simulink model "nav_leha19b"  (R2019b)
settings: Solver=FixedStepDiscrete  StartTime=0.0  StopTime=2500  FixedStep=dT  RelTol=1e-3
values from neighbouring files (symbols this model uses):
  al_gp_M = k    (= 2)    [gnss_data_orig.m]
  al_gp_max = 15    [model_nav_system_flight_simulation_orig.m]
  al_gp_mu = 3.986004418E+14    (= 398600441800000)    [gnss_data_orig.m]
  al_gp_resolution = 1000    [gnss_data_orig.m]
  al_gp_t0 = gnss_strings_2(1,4)    [gnss_data_orig.m]
  dT = 1    [model_nav_system_flight_simulation_orig.m]
  mean_p_ion = 1.3    [model_nav_system_flight_simulation_orig.m]
  mean_p_trop = 0.3    [model_nav_system_flight_simulation_orig.m]
  P0_b_g = zeros(23,23)    [model_nav_system_flight_simulation_orig.m]
  P_b = zeros(21, 21)    [model_nav_system_flight_simulation_orig.m]
  R_a = 6378136    [model_nav_system_flight_simulation_orig.m]
  R_betta = 0.0053171    [model_nav_system_flight_simulation_orig.m]
  R_betta1 = 71 * 10^-7    (= 7.1e-06)    [model_nav_system_flight_simulation_orig.m]
  R_e2 = 0    [model_nav_system_flight_simulation_orig.m]
  R_ge = 9.78049    [model_nav_system_flight_simulation_orig.m]
  R_q = 0.00346775    [model_nav_system_flight_simulation_orig.m]
  R_u = 7.292115*10^(-5)    (= 7.292115e-05)    [model_nav_system_flight_simulation_orig.m]
  sigma_error_acs0 = [SKO_del_n_x SKO_del_n_y SKO_del_n_z]    [model_nav_system_flight_simulation_orig.m]
  sigma_error_DUS0 = [SKO_del_Omega_x SKO_del_Omega_y SKO_del_Omega_z]    [model_nav_system_flight_simulation_orig.m]
  sigma_gnss0 = SKO_p_del_T + SKO_p_del_t + mean_p_ion + mean_p_trop + SKO_p_mnogoluch + SKO_p_noise    (= 5.61)    [model_nav_system_flight_simulation_orig.m]
  SKO_p_del_T = 3    [model_nav_system_flight_simulation_orig.m]
  SKO_p_del_t = 0.01    [model_nav_system_flight_simulation_orig.m]
  SKO_p_mnogoluch = 0.5    [model_nav_system_flight_simulation_orig.m]
  SKO_p_noise = 0.5    [model_nav_system_flight_simulation_orig.m]
  tr_H = flight_mission(3,1)    [model_nav_system_flight_simulation_orig.m]
  W = W'    [model_nav_system_flight_simulation_orig.m]
  X0 = X0'    [model_nav_system_flight_simulation_orig.m]
  X0_b_g = X0_b_g * 0    [model_nav_system_flight_simulation_orig.m]
undefined symbols (not defined in the file or in its folder): al_gp_e, al_gp_health, al_gp_i, al_gp_lan, al_gp_m0, al_gp_sqrt_a, al_gp_w, sigma_error_D_p, sigma_error_D_p1, sigma_gnss0_0, tr_course, tr_fi, tr_la, tr_pitch, tr_roll, tr_V_E, tr_V_H, tr_V_N, tr_X_dgsk, tr_Y_dgsk, tr_Z_dgsk
libraries: simulink_extras x8
(part 1 of 3)
settings Model: PacingRate=11  Creator=Алексей  LastModifiedBy=ssa33
settings DebuggingCC: ReadBeforeWriteMsg=DisableAll  WriteAfterWriteMsg=DisableAll  WriteAfterReadMsg=DisableAll  MultiTaskDSMMsg=none  ArithmeticOperatorsInVariantConditions=warning
settings ModelReferenceCC: UpdateModelReferenceTargets=IfOutOfDate
settings SFSimCC: SFSimEcho=off  CustomCodeUndefinedFunction=UseInterfaceOnly

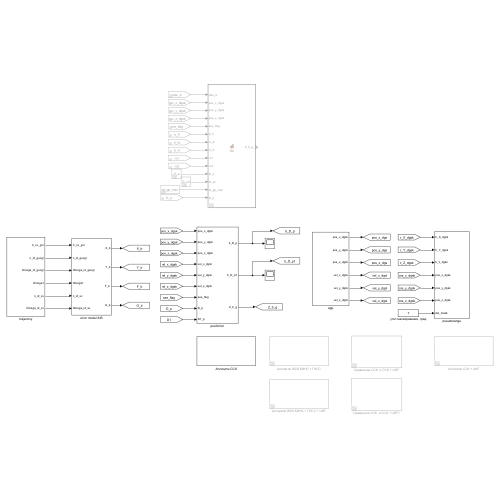
[thumbnail: Simulink's stored preview of the top-level diagram]
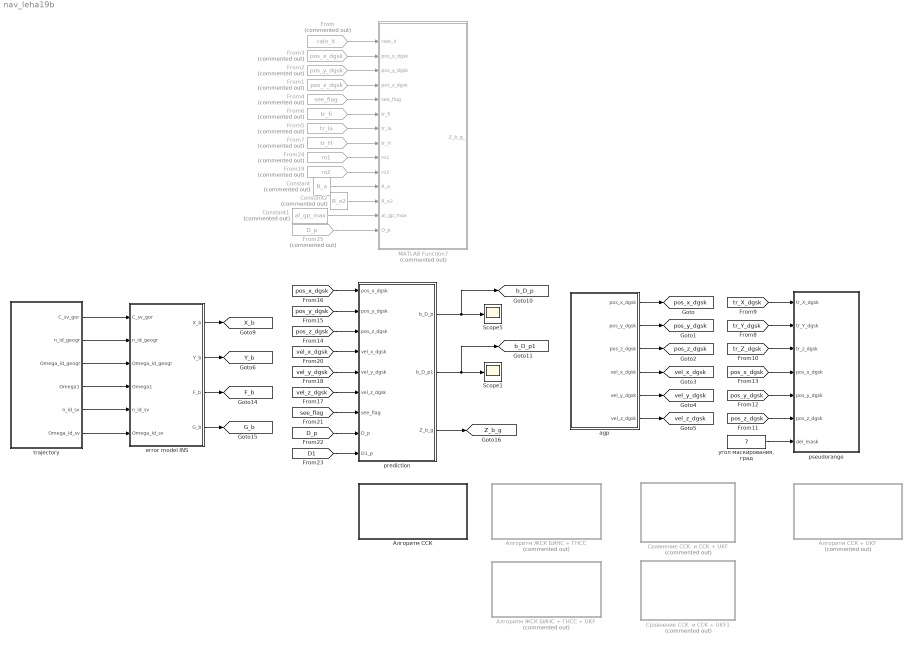
== system nav_leha19b ==
  Constant : Constant  Commented=on  Value=R_a
  Constant1 : Constant  Commented=on  Value=al_gp_max
  Constant2 : Constant  Commented=on  Value=R_e2
  From : From  Commented=on  GotoTag=rate_X  TagVisibility=global
  From1 : From  Commented=on  GotoTag=pos_z_dgsk  TagVisibility=global
  From19 : From  Commented=on  GotoTag=ro2  TagVisibility=global
  From2 : From  Commented=on  GotoTag=pos_y_dgsk  TagVisibility=global
  From24 : From  Commented=on  GotoTag=ro1  TagVisibility=global
  From25 : From  Commented=on  GotoTag=D_p  TagVisibility=global
  From3 : From  Commented=on  GotoTag=pos_x_dgsk  TagVisibility=global
  From4 : From  Commented=on  GotoTag=see_flag  TagVisibility=global
  From5 : From  Commented=on  GotoTag=tr_la  TagVisibility=global
  From6 : From  Commented=on  GotoTag=tr_fi  TagVisibility=global
  From7 : From  Commented=on  GotoTag=tr_H  TagVisibility=global
  MATLAB Function7 : MATLAB Function  Commented=on  TreatAsAtomicUnit=on
  Scope1 : Scope
  Scope5 : Scope
  agp : Subsystem
  error model INS : Subsystem
  "prediction " : Subsystem
  pseudorange : Subsystem
  trajectory : Subsystem
  Алгоритм ЖСК БИНС + ГНСС : Subsystem  Commented=on
  Алгоритм ЖСК БИНС + ГНСС + UKF : Subsystem  Commented=on
  Алгоритм ССК : Subsystem
  Алгоритм ССК + UKF : Subsystem  Commented=on
  Сравнение ССK  и CCK + UKF : Subsystem  Commented=on
  Сравнение ССK  и CCK + UKF1 : Subsystem  Commented=on
  "угол маскирования, град" : Constant  Value=7
  tag scope: F_b=global, G_b=global, X_b=global, Y_b=global, Z_b_g=global, b_D_p1=global, b_D_p=global, pos_x_dgsk=global, pos_y_dgsk=global, pos_z_dgsk=global, vel_x_dgsk=global, vel_y_dgsk=global, vel_z_dgsk=global
  wires:
  agp/1(pos_x_dgsk) -> [pos_x_dgsk]
  agp/2(pos_y_dgsk) -> [pos_y_dgsk]
  agp/3(pos_z_dgsk) -> [pos_z_dgsk]
  [tr_X_dgsk] -> pseudorange/1(tr_X_dgsk)
  [tr_Y_dgsk] -> pseudorange/2(tr_Y_dgsk)
  [tr_Z_dgsk] -> pseudorange/3(tr_z_dgsk)
  [pos_x_dgsk] -> pseudorange/4(pos_x_dgsk)
  [pos_y_dgsk] -> pseudorange/5(pos_y_dgsk)
  [pos_z_dgsk] -> pseudorange/6(pos_z_dgsk)
  "угол маскирования, град"/1 -> pseudorange/7(del_mask)
  agp/4(vel_x_dgsk) -> [vel_x_dgsk]
  agp/5(vel_y_dgsk) -> [vel_y_dgsk]
  agp/6(vel_z_dgsk) -> [vel_z_dgsk]
  error model INS/2(Y_b) -> [Y_b]
  [pos_x_dgsk] -> "prediction "/1(pos_x_dgsk)
  [pos_z_dgsk] -> "prediction "/3(pos_z_dgsk)
  [pos_y_dgsk] -> "prediction "/2(pos_y_dgsk)
  [vel_y_dgsk] -> "prediction "/5(vel_y_dgsk)
  [vel_z_dgsk] -> "prediction "/6(vel_z_dgsk)
  [vel_x_dgsk] -> "prediction "/4(vel_x_dgsk)
  "prediction "/1(b_D_p) -> [b_D_p], Scope5/1
  "prediction "/2(b_D_p1) -> [b_D_p1], Scope1/1
  [see_flag] -> "prediction "/7(see_flag)
  [D_p] -> "prediction "/8(D_p)
  [D1] -> "prediction "/9(D1_p)
  error model INS/1(X_b) -> [X_b]
  error model INS/3("F_b ") -> [F_b]
  error model INS/4(G_b) -> [G_b]
  trajectory/5(n_id_sv) -> error model INS/5(n_id_sv)
  trajectory/1(C_sv_gor) -> error model INS/1(C_sv_gor)
  trajectory/4(Omega1) -> error model INS/4(Omega1)
  trajectory/6(Omega_id_sv) -> error model INS/6(Omega_id_sv)
  trajectory/2(n_id_geogr) -> error model INS/2(n_id_geogr)
  trajectory/3(Omega_id_geogr) -> error model INS/3(Omega_id_geogr)
  From3/1 -> MATLAB Function7/2(pos_x_dgsk)
  From2/1 -> MATLAB Function7/3(pos_y_dgsk)
  From1/1 -> MATLAB Function7/4(pos_z_dgsk)
  From4/1 -> MATLAB Function7/5(see_flag)
  From6/1 -> MATLAB Function7/6(tr_fi)
  From5/1 -> MATLAB Function7/7(tr_la)
  From7/1 -> MATLAB Function7/8(tr_H)
  From24/1 -> MATLAB Function7/9(ro1)
  From19/1 -> MATLAB Function7/10(ro2)
  Constant/1 -> MATLAB Function7/11(R_a)
  Constant2/1 -> MATLAB Function7/12(R_e2)
  Constant1/1 -> MATLAB Function7/13(al_gp_max)
  From25/1 -> MATLAB Function7/14(D_p)
  From/1 -> MATLAB Function7/1(rate_X)
  "prediction "/3(Z_b_g) -> [Z_b_g]

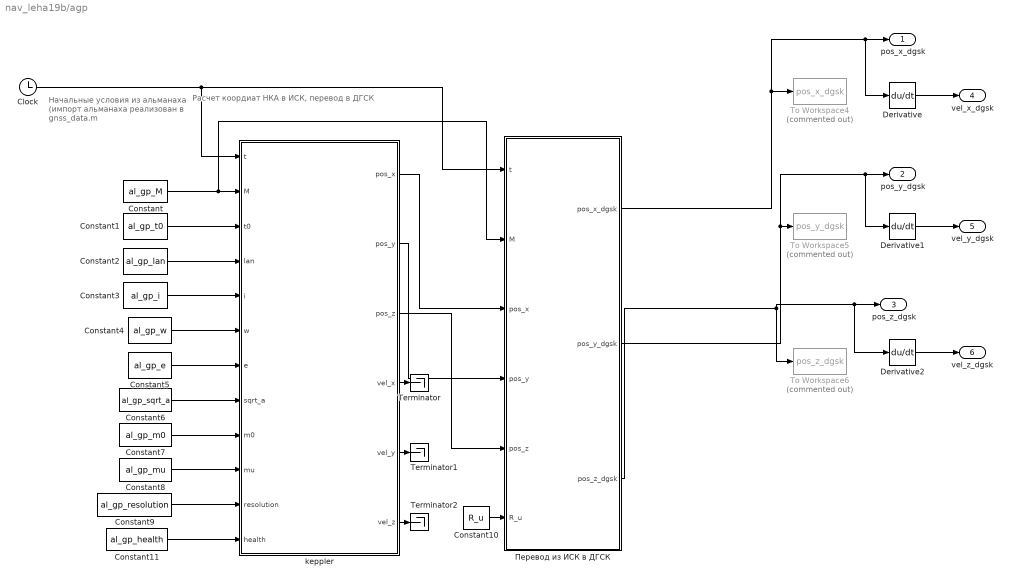
== system nav_leha19b/agp ==
  note: Начальные условия
      | из альманаха
      | (импорт альманаха
      | реализован в gnss_data.m
  note: Расчет коордиат НКА в ИСК, перевод в ДГСК
  Clock : Clock
  Constant : Constant  Value=al_gp_M
  Constant1 : Constant  Value=al_gp_t0
  Constant10 : Constant  Value=R_u
  Constant11 : Constant  Value=al_gp_health
  Constant2 : Constant  Value=al_gp_lan
  Constant3 : Constant  Value=al_gp_i
  Constant4 : Constant  Value=al_gp_w
  Constant5 : Constant  Value=al_gp_e
  Constant6 : Constant  Value=al_gp_sqrt_a
  Constant7 : Constant  Value=al_gp_m0
  Constant8 : Constant  Value=al_gp_mu
  Constant9 : Constant  Value=al_gp_resolution
  Derivative : Derivative
  Derivative1 : Derivative
  Derivative2 : Derivative
  Terminator : Terminator
  Terminator1 : Terminator
  Terminator2 : Terminator
  To Workspace4 : ToWorkspace  Commented=on  VariableName=pos_x_dgsk  SampleTime=-1
      settings: Save2DSignal=2-D array (concatenate along first dimension)
  To Workspace5 : ToWorkspace  Commented=on  VariableName=pos_y_dgsk  SampleTime=-1
      settings: Save2DSignal=2-D array (concatenate along first dimension)
  To Workspace6 : ToWorkspace  Commented=on  VariableName=pos_z_dgsk  SampleTime=-1
      settings: Save2DSignal=2-D array (concatenate along first dimension)
  keppler : MATLAB Function  TreatAsAtomicUnit=on
  Перевод из ИСК в ДГСК : MATLAB Function  TreatAsAtomicUnit=on
  pos_x_dgsk : Outport  VectorParamsAs1DForOutWhenUnconnected=off
  pos_y_dgsk : Outport  Port=2  VectorParamsAs1DForOutWhenUnconnected=off
  pos_z_dgsk : Outport  Port=3  VectorParamsAs1DForOutWhenUnconnected=off
  vel_x_dgsk : Outport  Port=4  VectorParamsAs1DForOutWhenUnconnected=off
  vel_y_dgsk : Outport  Port=5  VectorParamsAs1DForOutWhenUnconnected=off
  vel_z_dgsk : Outport  Port=6  VectorParamsAs1DForOutWhenUnconnected=off
  wires:
  Constant6/1 -> keppler/8(sqrt_a)
  Constant3/1 -> keppler/5(i)
  Constant10/1 -> Перевод из ИСК в ДГСК/6(R_u)
  Constant/1 -> Перевод из ИСК в ДГСК/2(M), keppler/2(M)
  Constant5/1 -> keppler/7(e)
  Constant2/1 -> keppler/4(lan)
  Constant8/1 -> keppler/10(mu)
  Constant7/1 -> keppler/9(m0)
  Constant11/1 -> keppler/12(health)
  Constant1/1 -> keppler/3(t0)
  Constant9/1 -> keppler/11(resolution)
  Constant4/1 -> keppler/6(w)
  Перевод из ИСК в ДГСК/3(pos_z_dgsk) -> To Workspace6/1, Derivative2/1, pos_z_dgsk/1
  Перевод из ИСК в ДГСК/2(pos_y_dgsk) -> Derivative1/1, pos_y_dgsk/1, To Workspace5/1
  Перевод из ИСК в ДГСК/1(pos_x_dgsk) -> To Workspace4/1, Derivative/1, pos_x_dgsk/1
  Clock/1 -> Перевод из ИСК в ДГСК/1(t), keppler/1(t)
  Derivative2/1 -> vel_z_dgsk/1
  Derivative/1 -> vel_x_dgsk/1
  Derivative1/1 -> vel_y_dgsk/1
  keppler/1(pos_x) -> Перевод из ИСК в ДГСК/3(pos_x)
  keppler/2(pos_y) -> Перевод из ИСК в ДГСК/4(pos_y)
  keppler/3(pos_z) -> Перевод из ИСК в ДГСК/5(pos_z)
  keppler/4(vel_x) -> Terminator/1
  keppler/5(vel_y) -> Terminator1/1
  keppler/6(vel_z) -> Terminator2/1

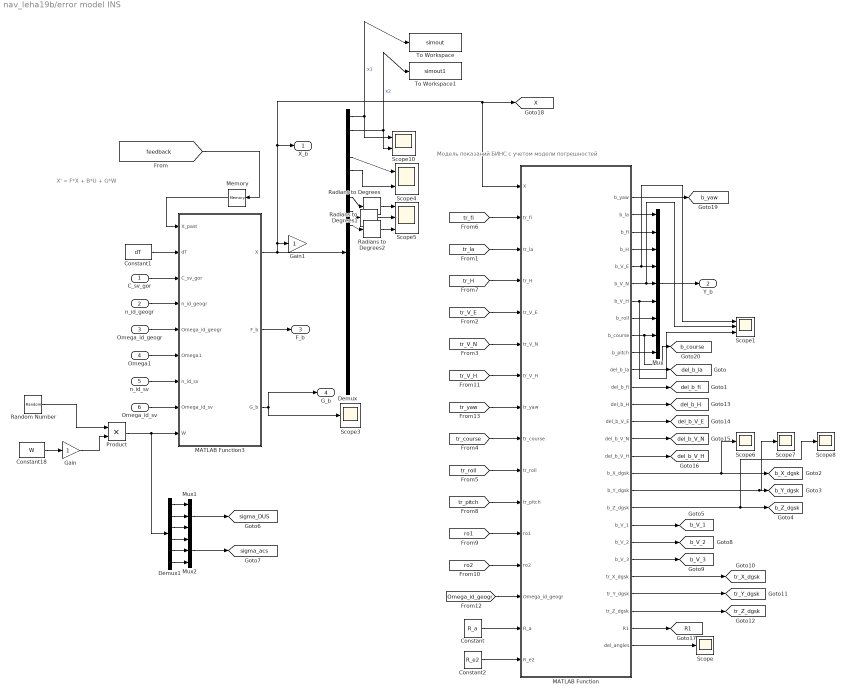
== system nav_leha19b/error model INS ==
  note: Модель показаний БИНС с учетом модели погрешностей
  note: X' = F*X + B*U + G*W
  C_sv_gor : Inport
  n_id_geogr : Inport  Port=2
  Omega_id_geogr : Inport  Port=3
  Omega1 : Inport  Port=4
  n_id_sv : Inport  Port=5
  Omega_id_sv : Inport  Port=6
  Constant : Constant  Value=R_a
  Constant1 : Constant  Value=dT
  Constant18 : Constant  Value=W  SampleTime=dT
  Constant2 : Constant  Value=R_e2
  Demux : Demux  Outputs=21
  Demux1 : Demux  Outputs=6
  Gain : Gain
  Gain1 : Gain
  MATLAB Function : MATLAB Function  TreatAsAtomicUnit=on
  MATLAB Function3 : MATLAB Function  TreatAsAtomicUnit=on
  Memory : Memory  InitialCondition=X0
  Mux : Mux  Inputs=9
  Mux1 : Mux  Inputs=3
  Mux2 : Mux  Inputs=3
  Product : Product
  Radians to Degrees : simulink_extras/Transformations/Radians to Degrees
  Radians to Degrees1 : simulink_extras/Transformations/Radians to Degrees
  Radians to Degrees2 : simulink_extras/Transformations/Radians to Degrees
  Random Number : RandomNumber
  Scope{,3,6..8} (5 alike) : Scope
  Scope1 : Scope  NumInputPorts=3
  Scope10 : Scope  NumInputPorts=2
  Scope4 : Scope  NumInputPorts=2
  Scope5 : Scope  NumInputPorts=3
  To Workspace : ToWorkspace  VariableName=simout  SampleTime=-1
      settings: Save2DSignal=2-D array (concatenate along first dimension)
  To Workspace1 : ToWorkspace  VariableName=simout1  SampleTime=-1
      settings: Save2DSignal=2-D array (concatenate along first dimension)
  X_b : Outport  VectorParamsAs1DForOutWhenUnconnected=off
  Y_b : Outport  Port=2  VectorParamsAs1DForOutWhenUnconnected=off
  "F_b " : Outport  Port=3  VectorParamsAs1DForOutWhenUnconnected=off
  G_b : Outport  Port=4  VectorParamsAs1DForOutWhenUnconnected=off
  tag scope: R1=global, X=global, b_V_1=global, b_V_2=global, b_V_3=global, b_X_dgsk=global, b_Y_dgsk=global, b_Z_dgsk=global, b_course=global, b_yaw=global, del_b_H=global, del_b_V_E=global, del_b_V_H=global, del_b_V_N=global, del_b_fi=global, del_b_la=global, sigma_DUS=global, sigma_acs=global, tr_X_dgsk=global, tr_Y_dgsk=global, tr_Z_dgsk=global
  wires:
  Constant1/1 -> MATLAB Function3/2(dT)
  Demux/9 -> Radians to Degrees2/1
  Demux/8 -> Radians to Degrees1/1
  Demux/7 -> Radians to Degrees/1
  Random Number/1 -> Product/1
  Product/1 -> MATLAB Function3/9(W), Demux1/1
  Constant18/1 -> Gain/1
  C_sv_gor/1 -> MATLAB Function3/3(C_sv_gor)
  n_id_geogr/1 -> MATLAB Function3/4(n_id_geogr)
  Omega_id_geogr/1 -> MATLAB Function3/5(Omega_id_geogr)
  Omega1/1 -> MATLAB Function3/6(Omega1)
  n_id_sv/1 -> MATLAB Function3/7(n_id_sv)
  Omega_id_sv/1 -> MATLAB Function3/8(Omega_id_sv)
  [tr_fi] -> MATLAB Function/2(tr_fi)
  [tr_H] -> MATLAB Function/4(tr_H)
  [tr_la] -> MATLAB Function/3(tr_la)
  [tr_V_E] -> MATLAB Function/5(tr_V_E)
  [tr_V_N] -> MATLAB Function/6(tr_V_N)
  [tr_course] -> MATLAB Function/9(tr_course)
  [tr_roll] -> MATLAB Function/10(tr_roll)
  [tr_pitch] -> MATLAB Function/11(tr_pitch)
  [ro1] -> MATLAB Function/12(ro1)
  [ro2] -> MATLAB Function/13(ro2)
  [Omega_id_geogr] -> MATLAB Function/14(Omega_id_geogr)
  [tr_V_H] -> MATLAB Function/7(tr_V_H)
  MATLAB Function/2(b_la) -> Mux/1
  MATLAB Function/3(b_fi) -> Mux/2
  MATLAB Function/4(b_H) -> Mux/3
  MATLAB Function/5(b_V_E) -> Scope1/1, Mux/4
  MATLAB Function/6(b_V_N) -> Scope1/2, Mux/5
  MATLAB Function/7(b_V_H) -> Scope1/3, Mux/6
  MATLAB Function/8(b_roll) -> Mux/7
  MATLAB Function/9(b_course) -> [b_course], Mux/8
  MATLAB Function/10(b_pitch) -> Mux/9
  Mux/1 -> Y_b/1
  Gain/1 -> Product/2
  MATLAB Function/11(del_b_la) -> [del_b_la]
  MATLAB Function/12(del_b_fi) -> [del_b_fi]
  MATLAB Function3/2(F_b) -> "F_b "/1
  Demux1/5 -> Mux2/2
  Demux1/4 -> Mux2/1
  Demux1/6 -> Mux2/3
  Demux1/1 -> Mux1/1
  Demux1/2 -> Mux1/2
  Demux1/3 -> Mux1/3
  Mux1/1 -> [sigma_DUS]
  Mux2/1 -> [sigma_acs]
  Constant2/1 -> MATLAB Function/16(R_e2)
  Constant/1 -> MATLAB Function/15(R_a)
  MATLAB Function/25(tr_Z_dgsk) -> [tr_Z_dgsk]
  MATLAB Function/24(tr_Y_dgsk) -> [tr_Y_dgsk]
  MATLAB Function/23(tr_X_dgsk) -> [tr_X_dgsk]
  MATLAB Function/22(b_V_3) -> [b_V_3]
  MATLAB Function/21(b_V_2) -> [b_V_2]
  MATLAB Function/20(b_V_1) -> [b_V_1]
  MATLAB Function/19(b_Z_dgsk) -> Scope8/1, [b_Z_dgsk]
  MATLAB Function/18(b_Y_dgsk) -> Scope7/1, [b_Y_dgsk]
  MATLAB Function/17(b_X_dgsk) -> Scope6/1, [b_X_dgsk]
  MATLAB Function/13(del_b_H) -> [del_b_H]
  MATLAB Function/15(del_b_V_N) -> [del_b_V_N]
  MATLAB Function/14(del_b_V_E) -> [del_b_V_E]
  MATLAB Function/16(del_b_V_H) -> [del_b_V_H]
  MATLAB Function/26(R1) -> [R1]
  Demux/2 -> To Workspace1/1, Scope10/2  "x2"
  MATLAB Function3/1(X) -> [X], MATLAB Function/1(X), X_b/1, Gain1/1, Demux/1
  [tr_yaw] -> MATLAB Function/8(tr_yaw)
  MATLAB Function/27(del_angles) -> Scope/1
  Demux/4 -> Scope4/1
  Demux/5 -> Scope4/2
  Demux/1 -> To Workspace/1, Scope10/1  "x1"
  MATLAB Function/1(b_yaw) -> [b_yaw]
  Memory/1 -> MATLAB Function3/1(X_past)
  MATLAB Function3/3(G_b) -> G_b/1, Scope3/1
  Radians to Degrees/1 -> Scope5/1
  Radians to Degrees1/1 -> Scope5/2
  Radians to Degrees2/1 -> Scope5/3
  [feedback] -> Memory/1

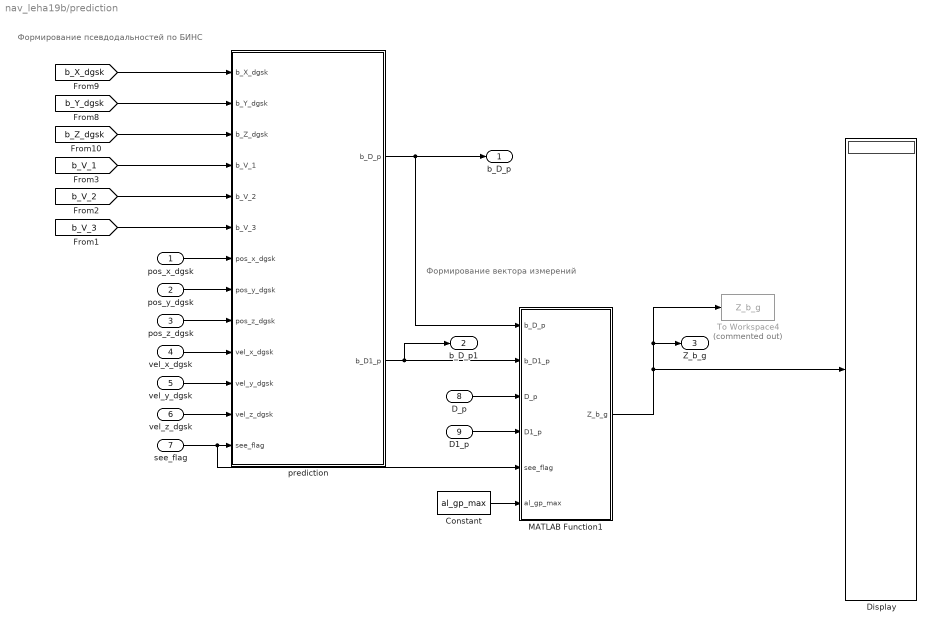
== system nav_leha19b/prediction  ==
  note: Формирование вектора измерений
  note: Формирование псевдодальностей по БИНС
  pos_x_dgsk : Inport
  pos_y_dgsk : Inport  Port=2
  pos_z_dgsk : Inport  Port=3
  vel_x_dgsk : Inport  Port=4
  vel_y_dgsk : Inport  Port=5
  vel_z_dgsk : Inport  Port=6
  see_flag : Inport  Port=7
  D_p : Inport  Port=8
  D1_p : Inport  Port=9
  Constant : Constant  Value=al_gp_max
  Display : Display
  MATLAB Function1 : MATLAB Function  TreatAsAtomicUnit=on
  To Workspace4 : ToWorkspace  Commented=on  VariableName=Z_b_g  SaveFormat=Structure  SampleTime=-1
      settings: Save2DSignal=2-D array (concatenate along first dimension)
  prediction : MATLAB Function  TreatAsAtomicUnit=on
  b_D_p : Outport  VectorParamsAs1DForOutWhenUnconnected=off
  b_D_p1 : Outport  Port=2  VectorParamsAs1DForOutWhenUnconnected=off
  Z_b_g : Outport  Port=3  VectorParamsAs1DForOutWhenUnconnected=off
  wires:
  [b_X_dgsk] -> prediction/1(b_X_dgsk)
  [b_Y_dgsk] -> prediction/2(b_Y_dgsk)
  [b_Z_dgsk] -> prediction/3(b_Z_dgsk)
  pos_x_dgsk/1 -> prediction/7(pos_x_dgsk)
  pos_y_dgsk/1 -> prediction/8(pos_y_dgsk)
  pos_z_dgsk/1 -> prediction/9(pos_z_dgsk)
  vel_x_dgsk/1 -> prediction/10(vel_x_dgsk)
  vel_y_dgsk/1 -> prediction/11(vel_y_dgsk)
  vel_z_dgsk/1 -> prediction/12(vel_z_dgsk)
  prediction/1(b_D_p) -> MATLAB Function1/1(b_D_p), b_D_p/1
  prediction/2(b_D1_p) -> b_D_p1/1, MATLAB Function1/2(b_D1_p)
  see_flag/1 -> MATLAB Function1/5(see_flag), prediction/13(see_flag)
  D_p/1 -> MATLAB Function1/3(D_p)
  D1_p/1 -> MATLAB Function1/4(D1_p)
  MATLAB Function1/1(Z_b_g) -> To Workspace4/1, Z_b_g/1, Display/1
  Constant/1 -> MATLAB Function1/6(al_gp_max)
  [b_V_1] -> prediction/4(b_V_1)
  [b_V_2] -> prediction/5(b_V_2)
  [b_V_3] -> prediction/6(b_V_3)

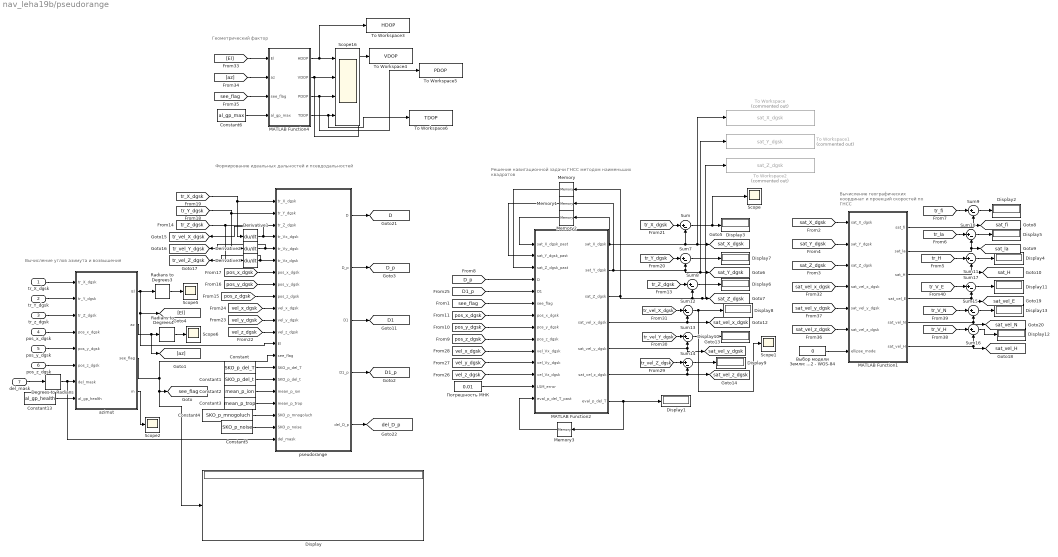
== system nav_leha19b/pseudorange ==
  note: Вычисление географических
      | координат и проекций
      | скоростей по ГНСС
  note: Решение навигационной задачи ГНСС методом
      | наименьших квадратов
  note: Геометрический фактор
  note: Формирование идеальных дальностей и
      | псевдодальностей
  note: Вычисление углов азимута и возвышения
  tr_X_dgsk : Inport
  tr_Y_dgsk : Inport  Port=2
  tr_z_dgsk : Inport  Port=3
  pos_x_dgsk : Inport  Port=4
  pos_y_dgsk : Inport  Port=5
  pos_z_dgsk : Inport  Port=6
  del_mask : Inport  Port=7
  Constant : Constant  Value=SKO_p_del_T
  Constant1 : Constant  Value=SKO_p_del_t
  Constant13 : Constant  Value=al_gp_health
  Constant2 : Constant  Value=mean_p_ion
  Constant3 : Constant  Value=mean_p_trop
  Constant4 : Constant  Value=SKO_p_mnogoluch
  Constant5 : Constant  Value=SKO_p_noise
  Constant6 : Constant  Value=al_gp_max
  Degrees to Radians : simulink_extras/Transformations/Degrees to Radians
  Derivative1 : Derivative
  Derivative2 : Derivative
  Derivative3 : Derivative
  Display{,1..13} (14 alike) : Display
  MATLAB Function1 : MATLAB Function  TreatAsAtomicUnit=on
  MATLAB Function2 : MATLAB Function  TreatAsAtomicUnit=on
  MATLAB Function4 : MATLAB Function  TreatAsAtomicUnit=on
  Memory : Memory
  Memory1 : Memory
  Memory2 : Memory
  Memory3 : Memory  InitialCondition=SKO_p_del_T
  Radians to Degrees3 : simulink_extras/Transformations/Radians to Degrees
  Radians to Degrees4 : simulink_extras/Transformations/Radians to Degrees
  Scope{,1..2,5..6} (5 alike) : Scope
  Scope16 : Scope  NumInputPorts=4
  Sum{,7..17} (12 alike) : Sum  Inputs=|+-
  To Workspace : ToWorkspace  Commented=on  VariableName=sat_X_dgsk  SampleTime=-1
  To Workspace1 : ToWorkspace  Commented=on  VariableName=sat_Y_dgsk  SampleTime=-1
  To Workspace2 : ToWorkspace  Commented=on  VariableName=sat_Z_dgsk  SampleTime=-1
  To Workspace3 : ToWorkspace  VariableName=HDOP  SampleTime=-1
      settings: Save2DSignal=2-D array (concatenate along first dimension)
  To Workspace4 : ToWorkspace  VariableName=VDOP  SampleTime=-1
      settings: Save2DSignal=2-D array (concatenate along first dimension)
  To Workspace5 : ToWorkspace  VariableName=PDOP  SampleTime=-1
      settings: Save2DSignal=2-D array (concatenate along first dimension)
  To Workspace6 : ToWorkspace  VariableName=TDOP  SampleTime=-1
      settings: Save2DSignal=2-D array (concatenate along first dimension)
  azimut : MATLAB Function  TreatAsAtomicUnit=on
  pseudorange : MATLAB Function  TreatAsAtomicUnit=on
  Выбор модели Земли: 0 - сфера 1 - ПЗ-90.11 2 - WGS-84 : Constant  Value=0
  Погрешность МНК : Constant  Value=0.01
  tag scope: D1=global, D1_p=global, D=global, D_p=global, del_D_p=global, sat_H=global, sat_X_dgsk=global, sat_Y_dgsk=global, sat_Z_dgsk=global, sat_fi=global, sat_la=global, sat_vel_E=global, sat_vel_H=global, sat_vel_N=global, sat_vel_x_dgsk=global, sat_vel_y_dgsk=global, sat_vel_z_dgsk=global, see_flag=global, tr_vel_X_dgsk=global, tr_vel_Y_dgsk=global, tr_vel_Z_dgsk=global
  wires:
  [tr_Z_dgsk] -> Derivative3/1, pseudorange/3(tr_Z_dgsk)
  [pos_z_dgsk] -> pseudorange/9(pos_z_dgsk)
  [pos_y_dgsk] -> pseudorange/8(pos_y_dgsk)
  [pos_x_dgsk] -> pseudorange/7(pos_x_dgsk)
  [tr_Y_dgsk] -> Derivative2/1, pseudorange/2(tr_Y_dgsk)
  azimut/2(az) -> [az], Radians to Degrees4/1
  [tr_X_dgsk] -> Derivative1/1, pseudorange/1(tr_X_dgsk)
  Degrees to Radians/1 -> pseudorange/21(del_mask), azimut/7(del_mask)
  tr_Y_dgsk/1 -> azimut/2(tr_Y_dgsk)
  Radians to Degrees3/1 -> Scope5/1
  Radians to Degrees4/1 -> Scope6/1
  azimut/1(El) -> [El], pseudorange/13(El), Radians to Degrees3/1
  del_mask/1 -> Degrees to Radians/1
  tr_z_dgsk/1 -> azimut/3(tr_Z_dgsk)
  pos_z_dgsk/1 -> azimut/6(pos_z_dgsk)
  pos_x_dgsk/1 -> azimut/4(pos_x_dgsk)
  pos_y_dgsk/1 -> azimut/5(pos_y_dgsk)
  tr_X_dgsk/1 -> azimut/1(tr_X_dgsk)
  Constant2/1 -> pseudorange/17(mean_p_ion)
  Constant3/1 -> pseudorange/18(mean_p_trop)
  Constant4/1 -> pseudorange/19(SKO_p_mnogoluch)
  Constant5/1 -> pseudorange/20(SKO_p_noise)
  Constant13/1 -> azimut/8(al_gp_health)
  azimut/4(m) -> Scope2/1
  [El] -> MATLAB Function4/1(El)
  [az] -> MATLAB Function4/2(az)
  [see_flag] -> MATLAB Function4/3(see_flag)
  MATLAB Function4/2(VDOP) -> Scope16/2, To Workspace4/1
  MATLAB Function4/3(PDOP) -> To Workspace5/1, Scope16/3
  Constant6/1 -> MATLAB Function4/4(al_gp_max)
  [tr_Z_dgsk] -> Sum8/1
  MATLAB Function2/2(sat_Y_dgsk) -> To Workspace1/1, [sat_Y_dgsk], Sum7/2, Memory1/1
  azimut/3(see_flag) -> [see_flag], Display/1, pseudorange/14(see_flag)
  [tr_Y_dgsk] -> Sum7/1
  [tr_X_dgsk] -> Sum/1
  MATLAB Function2/1(sat_X_dgsk) -> Memory2/1, Sum/2, To Workspace/1, [sat_X_dgsk]
  MATLAB Function2/3(sat_Z_dgsk) -> To Workspace2/1, [sat_Z_dgsk], Sum8/2, Memory/1
  [D_p] -> MATLAB Function2/4(D)
  Memory/1 -> MATLAB Function2/3(sat_Z_dgsk_past)
  Memory1/1 -> MATLAB Function2/2(sat_Y_dgsk_past)
  Memory2/1 -> MATLAB Function2/1(sat_X_dgsk_past)
  [pos_x_dgsk] -> MATLAB Function2/7(pos_x_dgsk)
  [pos_z_dgsk] -> MATLAB Function2/9(pos_z_dgsk)
  [pos_y_dgsk] -> MATLAB Function2/8(pos_y_dgsk)
  Sum/1 -> Scope/1, Display3/1
  Sum7/1 -> Display7/1
  Sum8/1 -> Display6/1
  MATLAB Function2/7(eval_p_del_T) -> Memory3/1, Display1/1
  [see_flag] -> MATLAB Function2/6(see_flag)
  Погрешность МНК/1 -> MATLAB Function2/13(LSM_error)
  Memory3/1 -> MATLAB Function2/14(eval_p_del_T_past)
  [sat_X_dgsk] -> MATLAB Function1/1(sat_X_dgsk)
  [sat_Y_dgsk] -> MATLAB Function1/2(sat_Y_dgsk)
  [sat_Z_dgsk] -> MATLAB Function1/3(sat_Z_dgsk)
  Sum11/1 -> Display4/1
  Sum10/1 -> Display5/1
  Sum9/1 -> Display2/1
  MATLAB Function1/3(sat_H) -> Sum11/2, [sat_H]
  MATLAB Function1/1(sat_fi) -> Sum9/2, [sat_fi]
  [tr_fi] -> Sum9/1
  [tr_la] -> Sum10/1
  MATLAB Function1/2(sat_la) -> Sum10/2, [sat_la]
  [tr_H] -> Sum11/1
  Выбор модели Земли: 0 - сфера 1 - ПЗ-90.11 2 - WGS-84/1 -> MATLAB Function1/7(ellipse_mode)
  Derivative1/1 -> [tr_vel_X_dgsk], pseudorange/4(tr_Vx_dgsk)
  Derivative2/1 -> [tr_vel_Y_dgsk], pseudorange/5(tr_Vy_dgsk)
  Derivative3/1 -> pseudorange/6(tr_Vz_dgsk), [tr_vel_Z_dgsk]
  pseudorange/3(D1) -> [D1]
  [vel_x_dgsk] -> pseudorange/10(vel_x_dgsk)
  [vel_y_dgsk] -> pseudorange/11(vel_y_dgsk)
  [vel_z_dgsk] -> pseudorange/12(vel_z_dgsk)
  [D1_p] -> MATLAB Function2/5(D1)
  [vel_x_dgsk] -> MATLAB Function2/10(vel_Vx_dgsk)
  [vel_y_dgsk] -> MATLAB Function2/11(vel_Vy_dgsk)
  [vel_z_dgsk] -> MATLAB Function2/12(vel_Vz_dgsk)
  Sum14/1 -> Display9/1
  Sum13/1 -> Display10/1
  Sum12/1 -> Display8/1, Scope1/1
  MATLAB Function2/6(sat_vel_z_dgsk) -> [sat_vel_z_dgsk], Sum14/2
  MATLAB Function2/4(sat_vel_x_dgsk) -> [sat_vel_x_dgsk], Sum12/2
  [tr_vel_X_dgsk] -> Sum12/1
  [tr_vel_Y_dgsk] -> Sum13/1
  MATLAB Function2/5(sat_vel_y_dgsk) -> [sat_vel_y_dgsk], Sum13/2
  [tr_vel_Z_dgsk] -> Sum14/1
  [sat_vel_x_dgsk] -> MATLAB Function1/4(sat_vel_x_dgsk)
  [sat_vel_y_dgsk] -> MATLAB Function1/5(sat_vel_y_dgsk)
  [sat_vel_z_dgsk] -> MATLAB Function1/6(sat_vel_z_dgsk)
  [tr_V_H] -> Sum16/1
  MATLAB Function1/5(sat_vel_N) -> Sum15/2, [sat_vel_N]
  [tr_V_N] -> Sum15/1
  [tr_V_E] -> Sum17/1
  MATLAB Function1/4(sat_vel_E) -> [sat_vel_E], Sum17/2
  MATLAB Function1/6(sat_vel_H) -> Sum16/2, [sat_vel_H]
  Sum17/1 -> Display11/1
  Sum15/1 -> Display13/1
  Sum16/1 -> Display12/1
  pseudorange/4(D1_p) -> [D1_p]
  pseudorange/2(D_p) -> [D_p]
  pseudorange/1(D) -> [D]
  Constant/1 -> pseudorange/15(SKO_p_del_T)
  Constant1/1 -> pseudorange/16(SKO_p_del_t)
  pseudorange/5(del_D_p) -> [del_D_p]
  MATLAB Function4/1(HDOP) -> To Workspace3/1, Scope16/1
  MATLAB Function4/4(TDOP) -> To Workspace6/1, Scope16/4

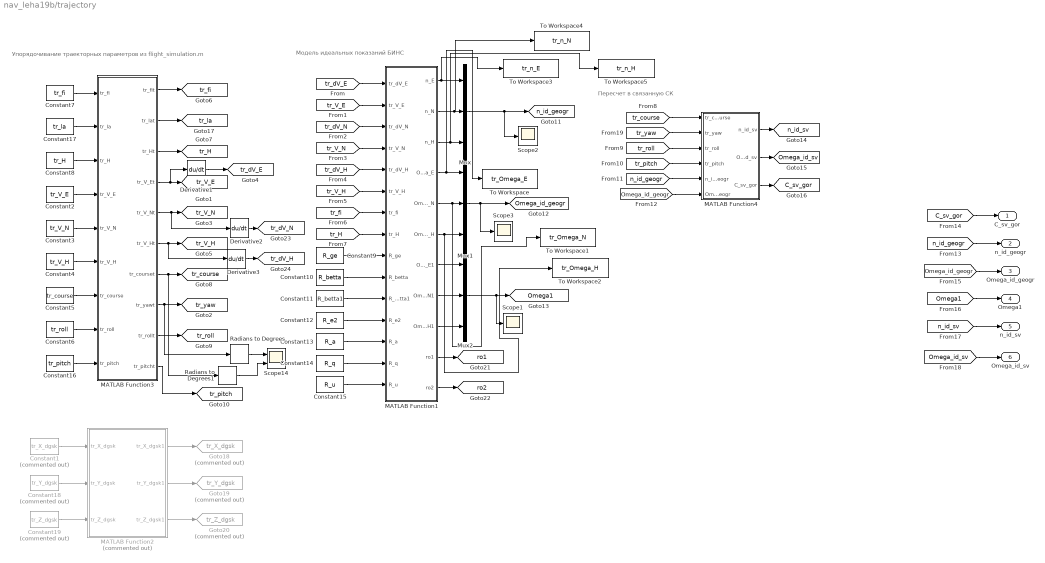
== system nav_leha19b/trajectory ==
  note: Пересчет в связанную СК
  note: Модель идеальных показаний БИНС
  note: Упорядочивание траекторных параметров из flight_simulation.m
  Constant1 : Constant  Commented=on  Value=tr_X_dgsk
  Constant10 : Constant  Value=R_betta
  Constant11 : Constant  Value=R_betta1
  Constant12 : Constant  Value=R_e2
  Constant13 : Constant  Value=R_a
  Constant14 : Constant  Value=R_q
  Constant15 : Constant  Value=R_u
  Constant16 : Constant  Value=tr_pitch
  Constant17 : Constant  Value=tr_la
  Constant18 : Constant  Commented=on  Value=tr_Y_dgsk
  Constant19 : Constant  Commented=on  Value=tr_Z_dgsk
  Constant2 : Constant  Value=tr_V_E
  Constant3 : Constant  Value=tr_V_N
  Constant4 : Constant  Value=tr_V_H
  Constant5 : Constant  Value=tr_course
  Constant6 : Constant  Value=tr_roll
  Constant7 : Constant  Value=tr_fi
  Constant8 : Constant  Value=tr_H
  Constant9 : Constant  Value=R_ge
  Derivative1 : Derivative
  Derivative2 : Derivative
  Derivative3 : Derivative
  Goto18 : Goto  Commented=on  GotoTag=tr_X_dgsk  TagVisibility=global
  Goto19 : Goto  Commented=on  GotoTag=tr_Y_dgsk  TagVisibility=global
  Goto20 : Goto  Commented=on  GotoTag=tr_Z_dgsk  TagVisibility=global
  MATLAB Function1 : MATLAB Function  TreatAsAtomicUnit=on
  MATLAB Function2 : MATLAB Function  Commented=on  TreatAsAtomicUnit=on
  MATLAB Function3 : MATLAB Function  TreatAsAtomicUnit=on
  MATLAB Function4 : MATLAB Function  TreatAsAtomicUnit=on
  Mux : Mux  Inputs=3
  Mux1 : Mux  Inputs=3
  Mux2 : Mux  Inputs=3
  Radians to Degrees : simulink_extras/Transformations/Radians to Degrees
  Radians to Degrees1 : simulink_extras/Transformations/Radians to Degrees
  Scope1 : Scope
  Scope14 : Scope  NumInputPorts=2
  Scope2 : Scope
  Scope3 : Scope
  To Workspace : ToWorkspace  VariableName=tr_Omega_E  SampleTime=-1
  To Workspace1 : ToWorkspace  VariableName=tr_Omega_N  SampleTime=-1
  To Workspace2 : ToWorkspace  VariableName=tr_Omega_H  SampleTime=-1
  To Workspace3 : ToWorkspace  VariableName=tr_n_E  SampleTime=-1
  To Workspace4 : ToWorkspace  VariableName=tr_n_N  SampleTime=-1
  To Workspace5 : ToWorkspace  VariableName=tr_n_H  SampleTime=-1
  C_sv_gor : Outport  VectorParamsAs1DForOutWhenUnconnected=off
  n_id_geogr : Outport  Port=2  VectorParamsAs1DForOutWhenUnconnected=off
  Omega_id_geogr : Outport  Port=3  VectorParamsAs1DForOutWhenUnconnected=off
  Omega1 : Outport  Port=4  VectorParamsAs1DForOutWhenUnconnected=off
  n_id_sv : Outport  Port=5  VectorParamsAs1DForOutWhenUnconnected=off
  Omega_id_sv : Outport  Port=6  VectorParamsAs1DForOutWhenUnconnected=off
  tag scope: C_sv_gor=global, Omega1=global, Omega_id_geogr=global, Omega_id_sv=global, n_id_geogr=global, n_id_sv=global, ro1=global, ro2=global, tr_H=global, tr_V_E=global, tr_V_H=global, tr_V_N=global, tr_course=global, tr_dV_E=global, tr_dV_H=global, tr_dV_N=global, tr_fi=global, tr_la=global, tr_pitch=global, tr_roll=global, tr_yaw=global
  wires:
  Constant4/1 -> MATLAB Function3/6(tr_V_H)
  Constant5/1 -> MATLAB Function3/7(tr_course)
  Constant2/1 -> MATLAB Function3/4(tr_V_E)
  [tr_V_H] -> MATLAB Function1/6(tr_V_H)
  [tr_course] -> MATLAB Function4/1(tr_course)
  Mux/1 -> Scope2/1, [n_id_geogr]
  MATLAB Function1/8(Omega1_N1) -> Mux2/2
  [tr_V_N] -> MATLAB Function1/4(tr_V_N)
  Constant16/1 -> MATLAB Function3/9(tr_pitch)
  Constant9/1 -> MATLAB Function1/9(R_ge)
  MATLAB Function4/1(n_id_sv) -> [n_id_sv]
  MATLAB Function1/9(Omega1_H1) -> Mux2/3
  Constant14/1 -> MATLAB Function1/14(R_q)
  [tr_dV_H] -> MATLAB Function1/5(tr_dV_H)
  [Omega_id_geogr] -> MATLAB Function4/6(Omega_id_geogr)
  MATLAB Function4/3(C_sv_gor) -> [C_sv_gor]
  MATLAB Function1/7(Omega1_E1) -> Mux2/1
  Radians to Degrees1/1 -> Scope14/2
  Constant13/1 -> MATLAB Function1/13(R_a)
  Constant15/1 -> MATLAB Function1/15(R_u)
  [tr_pitch] -> MATLAB Function4/4(tr_pitch)
  MATLAB Function1/5(Omega_N) -> To Workspace1/1, Mux1/2
  [tr_roll] -> MATLAB Function4/3(tr_roll)
  MATLAB Function1/2(n_N) -> To Workspace4/1, Mux/2
  MATLAB Function1/3(n_H) -> To Workspace5/1, Mux/3
  Constant17/1 -> MATLAB Function3/2(tr_la)
  Mux1/1 -> Scope3/1, [Omega_id_geogr]
  MATLAB Function1/4(Omega_E) -> To Workspace/1, Mux1/1
  Constant3/1 -> MATLAB Function3/5(tr_V_N)
  Constant6/1 -> MATLAB Function3/8(tr_roll)
  [tr_dV_E] -> MATLAB Function1/1(tr_dV_E)
  [tr_dV_N] -> MATLAB Function1/3(tr_dV_N)
  Mux2/1 -> Scope1/1, [Omega1]
  [tr_H] -> MATLAB Function1/8(tr_H)
  Constant12/1 -> MATLAB Function1/12(R_e2)
  [tr_V_E] -> MATLAB Function1/2(tr_V_E)
  Constant7/1 -> MATLAB Function3/1(tr_fi)
  MATLAB Function4/2(Omega_id_sv) -> [Omega_id_sv]
  MATLAB Function1/6(Omega_H) -> To Workspace2/1, Mux1/3
  [tr_fi] -> MATLAB Function1/7(tr_fi)
  Constant11/1 -> MATLAB Function1/11(R_betta1)
  Radians to Degrees/1 -> Scope14/1
  Constant8/1 -> MATLAB Function3/3(tr_H)
  MATLAB Function3/1(tr_fit) -> [tr_fi]
  [n_id_geogr] -> MATLAB Function4/5(n_id_geogr)
  MATLAB Function1/1(n_E) -> To Workspace3/1, Mux/1
  Constant10/1 -> MATLAB Function1/10(R_betta)
  [Omega1] -> Omega1/1
  [Omega_id_geogr] -> Omega_id_geogr/1
  [n_id_geogr] -> n_id_geogr/1
  [n_id_sv] -> n_id_sv/1
  [Omega_id_sv] -> Omega_id_sv/1
  [C_sv_gor] -> C_sv_gor/1
  MATLAB Function1/10(ro1) -> [ro1]
  MATLAB Function1/11(ro2) -> [ro2]
  MATLAB Function3/2(tr_lat) -> [tr_la]
  MATLAB Function3/3(tr_Ht) -> [tr_H]
  MATLAB Function3/4(tr_V_Et) -> Derivative1/1, [tr_V_E]
  MATLAB Function3/5(tr_V_Nt) -> Derivative2/1, [tr_V_N]
  MATLAB Function3/6(tr_V_Ht) -> Derivative3/1, [tr_V_H]
  MATLAB Function3/7(tr_courset) -> Radians to Degrees1/1, [tr_course]
  MATLAB Function3/9(tr_rollt) -> [tr_roll]
  MATLAB Function3/10(tr_pitcht) -> [tr_pitch]
  Constant1/1 -> MATLAB Function2/1(tr_X_dgsk)
  Constant18/1 -> MATLAB Function2/2(tr_Y_dgsk)
  Constant19/1 -> MATLAB Function2/3(tr_Z_dgsk)
  MATLAB Function2/1(tr_X_dgsk1) -> Goto18/1
  MATLAB Function2/2(tr_Y_dgsk1) -> Goto19/1
  MATLAB Function2/3(tr_Z_dgsk1) -> Goto20/1
  MATLAB Function3/8(tr_yawt) -> [tr_yaw], Radians to Degrees/1
  [tr_yaw] -> MATLAB Function4/2(tr_yaw)
  Derivative1/1 -> [tr_dV_E]
  Derivative3/1 -> [tr_dV_H]
  Derivative2/1 -> [tr_dV_N]

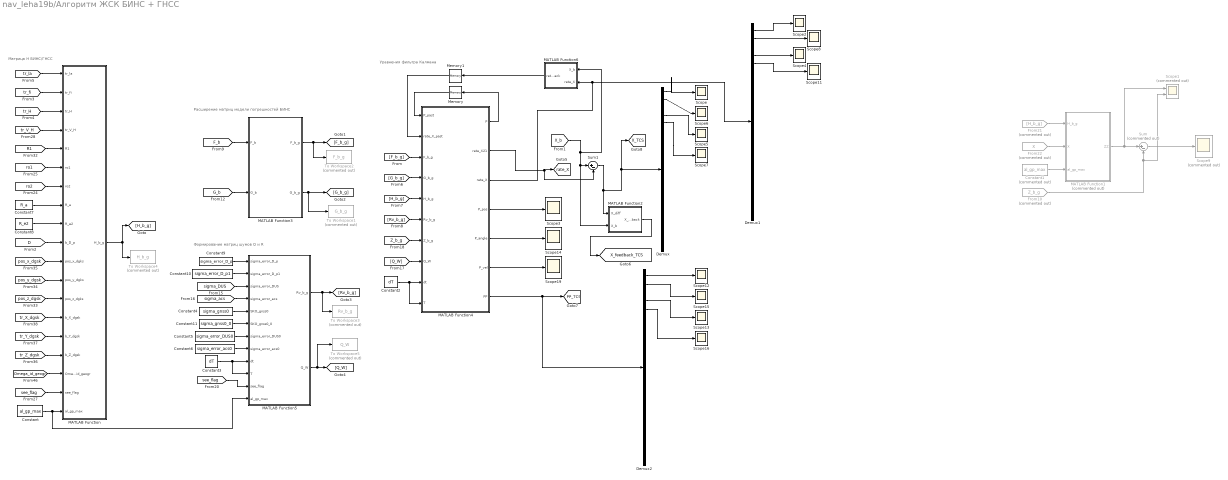
== system nav_leha19b/Алгоритм ЖСК БИНС + ГНСС ==
  note: Уравнения фильтра Калмана
  note: Формирование матриц шумов Q и R
  note: Расширение матриц модели погрешностей БИНС
  note: Матрица H БИНС/ГНСС
  Constant : Constant  Value=al_gp_max
  Constant1 : Constant  Commented=on  Value=al_gp_max
  Constant10 : Constant  Value=sigma_error_D_p1
  Constant11 : Constant  Value=sigma_gnss0_0
  Constant2 : Constant  Value=dT
  Constant3 : Constant  Value=dT
  Constant4 : Constant  Value=sigma_gnss0
  Constant5 : Constant  Value=sigma_error_DUS0
  Constant6 : Constant  Value=sigma_error_acs0
  Constant7 : Constant  Value=R_a
  Constant8 : Constant  Value=R_e2
  Constant9 : Constant  Value=sigma_error_D_p
  Demux : Demux  Outputs=21
  Demux1 : Demux  Outputs=23
  Demux2 : Demux  Outputs=23
  From10 : From  Commented=on  GotoTag=Z_b_g  TagVisibility=global
  From21 : From  Commented=on  GotoTag=H_b_g
  From22 : From  Commented=on  GotoTag=X  TagVisibility=global
  MATLAB Function : MATLAB Function  TreatAsAtomicUnit=on
  MATLAB Function1 : MATLAB Function  Commented=on  TreatAsAtomicUnit=on
  MATLAB Function2 : MATLAB Function  TreatAsAtomicUnit=on
  MATLAB Function3 : MATLAB Function  TreatAsAtomicUnit=on
  MATLAB Function4 : MATLAB Function  TreatAsAtomicUnit=on
  MATLAB Function5 : MATLAB Function  TreatAsAtomicUnit=on
  MATLAB Function6 : MATLAB Function  TreatAsAtomicUnit=on
  Memory : Memory  InitialCondition=P0_b_g
  Memory1 : Memory  InitialCondition=X0_b_g
  Scope{,2..8,11..16,19} (15 alike) : Scope
  Scope1 : Scope  Commented=on  NumInputPorts=2
  Scope9 : Scope  Commented=on
  Sum : Sum  Commented=on  Inputs=|+-
  Sum1 : Sum  Inputs=|+-
  To Workspace1 : ToWorkspace  Commented=on  VariableName=G_b_g  SaveFormat=Structure  SampleTime=-1
      settings: Save2DSignal=2-D array (concatenate along first dimension)
  To Workspace2 : ToWorkspace  Commented=on  VariableName=F_b_g  SaveFormat=Structure  SampleTime=-1
      settings: Save2DSignal=2-D array (concatenate along first dimension)
  To Workspace3 : ToWorkspace  Commented=on  VariableName=Rv_b_g  SaveFormat=Structure  SampleTime=-1
      settings: Save2DSignal=2-D array (concatenate along first dimension)
  To Workspace4 : ToWorkspace  Commented=on  VariableName=H_b_g  SaveFormat=Structure With Time  SampleTime=-1
  To Workspace5 : ToWorkspace  Commented=on  VariableName=Q_W  SaveFormat=Structure  SampleTime=-1
      settings: Save2DSignal=2-D array (concatenate along first dimension)
  tag scope: PP_TCS=global, X_TCS=global, X_feedback_TCS=global, rate_X=global
  wires:
  [Omega_id_geogr] -> MATLAB Function/17(Omega_id_geogr)
  Constant8/1 -> MATLAB Function/9(R_e2)
  [pos_y_dgsk] -> MATLAB Function/12(pos_y_dgks)
  MATLAB Function/1(H_b_g) -> To Workspace4/1, [H_b_g]
  [ro2] -> MATLAB Function/7(ro2)
  [tr_X_dgsk] -> MATLAB Function/14(b_X_dgsk)
  [ro1] -> MATLAB Function/6(ro1)
  [tr_Y_dgsk] -> MATLAB Function/15(b_Y_dgsk)
  [pos_x_dgsk] -> MATLAB Function/11(pos_x_dgks)
  [pos_z_dgsk] -> MATLAB Function/13(pos_z_dgks)
  [D] -> MATLAB Function/10(b_D_p)
  [tr_Z_dgsk] -> MATLAB Function/16(b_Z_dgsk)
  [R1] -> MATLAB Function/5(R1)
  Constant7/1 -> MATLAB Function/8(R_a)
  [F_b] -> MATLAB Function3/1(F_b)
  [G_b] -> MATLAB Function3/2(G_b)
  Constant2/1 -> MATLAB Function4/10(T), MATLAB Function4/9(dt)
  Constant9/1 -> MATLAB Function5/1(sigma_error_D_p)
  Constant10/1 -> MATLAB Function5/2(sigma_error_D_p1)
  [sigma_DUS] -> MATLAB Function5/3(sigma_error_DUS)
  [sigma_acs] -> MATLAB Function5/4(sigma_error_acs)
  Constant3/1 -> MATLAB Function5/10(T), MATLAB Function5/9(dt)
  MATLAB Function3/1(F_b_g) -> [F_b_g], To Workspace2/1
  MATLAB Function4/1(P) -> Memory/1
  MATLAB Function3/2(G_b_g) -> To Workspace1/1, [G_b_g]
  MATLAB Function5/1(Rv_b_g) -> [Rv_b_g], To Workspace3/1
  MATLAB Function5/2(Q_W) -> To Workspace5/1, [Q_W]
  [F_b_g] -> MATLAB Function4/3(F_b_g)
  [G_b_g] -> MATLAB Function4/4(G_b_g)
  [H_b_g] -> MATLAB Function4/5(H_b_g)
  [Rv_b_g] -> MATLAB Function4/6(Rv_b_g)
  [Q_W] -> MATLAB Function4/8(Q_W)
  [Z_b_g] -> MATLAB Function4/7(Z_b_g)
  MATLAB Function4/3(rate_X) -> MATLAB Function6/2(rate_X), Demux1/1
  Memory1/1 -> MATLAB Function4/2(rate_X_past)
  Memory/1 -> MATLAB Function4/1(P_past)
  Constant4/1 -> MATLAB Function5/5(SKO_gnss0)
  Constant5/1 -> MATLAB Function5/7(sigma_error_DUS0)
  Constant6/1 -> MATLAB Function5/8(sigma_error_acs0)
  [see_flag] -> MATLAB Function/18(see_flag)
  Constant/1 -> MATLAB Function5/12(al_gp_max), MATLAB Function/19(al_gp_max)
  [see_flag] -> MATLAB Function5/11(see_flag)
  MATLAB Function4/4(P_pos) -> Scope3/1
  [X_b] -> MATLAB Function2/2(X_b), Sum1/1, MATLAB Function6/1(X_b)
  Sum1/1 -> Demux/1, [X_TCS], MATLAB Function2/1(X_diff)
  MATLAB Function4/2(rate_X21) -> Sum1/2, [rate_X]
  Demux/1 -> Scope/1
  Demux/4 -> Scope5/1
  From21/1 -> MATLAB Function1/1(H_b_g)
  From22/1 -> MATLAB Function1/2(X)
  [tr_fi] -> MATLAB Function/2(tr_fi)
  [tr_H] -> MATLAB Function/3(tr_H)
  [tr_V_H] -> MATLAB Function/4(tr_V_H)
  [tr_la] -> MATLAB Function/1(tr_la)
  MATLAB Function4/5(P_angle) -> Scope14/1
  MATLAB Function2/1(X_feedback) -> [X_feedback_TCS]
  Demux1/1 -> Scope2/1
  MATLAB Function4/6(P_vel) -> Scope19/1
  Constant1/1 -> MATLAB Function1/3(al_gp_max)
  MATLAB Function6/1(rate_X_feedback) -> Memory1/1
  MATLAB Function4/7(PP) -> Demux2/1, [PP_TCS]
  From10/1 -> Scope1/2, Sum/2
  MATLAB Function1/1(ZZ) -> Scope1/1, Sum/1
  Sum/1 -> Scope9/1
  Constant11/1 -> MATLAB Function5/6(SKO_gnss0_0)
  Demux1/4 -> Scope4/1
  Demux/2 -> Scope6/1
  Demux/5 -> Scope7/1
  Demux1/2 -> Scope8/1
  Demux1/5 -> Scope11/1
  Demux2/1 -> Scope12/1
  Demux2/2 -> Scope15/1
  Demux2/4 -> Scope13/1
  Demux2/5 -> Scope16/1

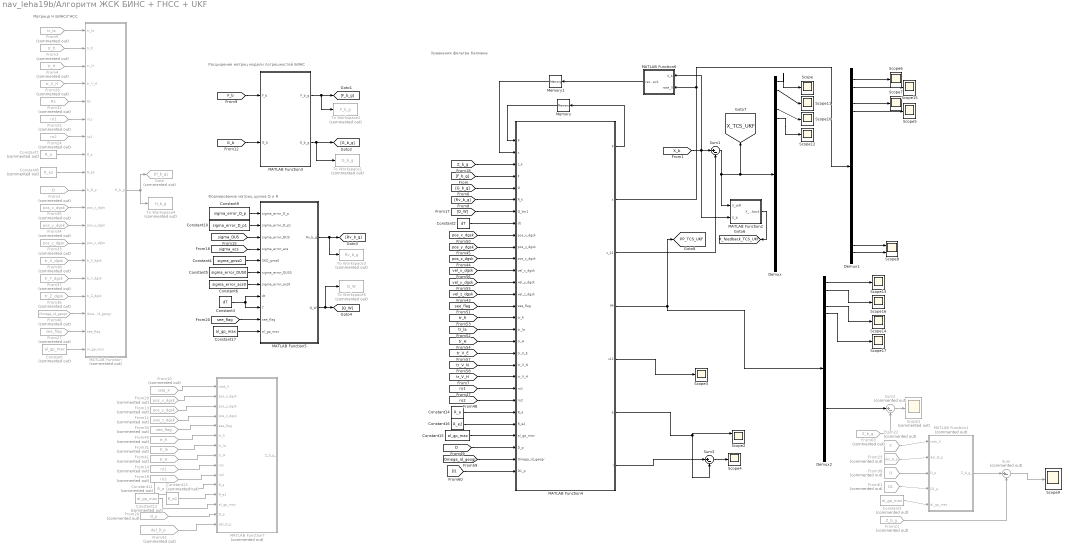
== system nav_leha19b/Алгоритм ЖСК БИНС + ГНСС + UKF ==
  note: Уравнения фильтра Калмана
  note: Формирование матриц шумов Q и R
  note: Расширение матриц модели погрешностей БИНС
  note: Матрица H БИНС/ГНСС
  Constant : Constant  Commented=on  Value=al_gp_max
  Constant1 : Constant  Commented=on  Value=al_gp_max
  Constant10 : Constant  Value=sigma_error_D_p1
  Constant11 : Constant  Commented=on  Value=R_a
  Constant12 : Constant  Commented=on  Value=al_gp_max
  Constant13 : Constant  Commented=on  Value=R_e2
  Constant14 : Constant  Value=R_a
  Constant15 : Constant  Value=al_gp_max
  Constant16 : Constant  Value=R_e2
  Constant17 : Constant  Value=al_gp_max
  Constant2 : Constant  Value=dT
  Constant3 : Constant  Value=dT
  Constant4 : Constant  Value=sigma_gnss0
  Constant5 : Constant  Value=sigma_error_DUS0
  Constant6 : Constant  Value=sigma_error_acs0
  Constant7 : Constant  Commented=on  Value=R_a
  Constant8 : Constant  Commented=on  Value=R_e2
  Constant9 : Constant  Value=sigma_error_D_p
  Demux : Demux  Outputs=21
  Demux1 : Demux  Outputs=23
  Demux2 : Demux  Outputs=23
  From10 : From  Commented=on  GotoTag=rate_X  TagVisibility=global
  From11 : From  Commented=on  GotoTag=pos_z_dgsk  TagVisibility=global
  From13 : From  Commented=on  GotoTag=pos_y_dgsk  TagVisibility=global
  From14 : From  Commented=on  GotoTag=ro1  TagVisibility=global
  From19 : From  Commented=on  GotoTag=ro2  TagVisibility=global
  From2 : From  Commented=on  GotoTag=D  TagVisibility=global
  From21 : From  Commented=on  GotoTag=Z_b_g  TagVisibility=global
  From22 : From  Commented=on  GotoTag=X  TagVisibility=global
  From23 : From  Commented=on  GotoTag=del_D_p  TagVisibility=global
  From24 : From  Commented=on  GotoTag=ro2  TagVisibility=global
  From25 : From  Commented=on  GotoTag=ro1  TagVisibility=global
  From26 : From  Commented=on  GotoTag=D_p  TagVisibility=global
  From27 : From  Commented=on  GotoTag=see_flag  TagVisibility=global
  From28 : From  Commented=on  GotoTag=tr_V_H  TagVisibility=global
  From29 : From  Commented=on  GotoTag=pos_x_dgsk  TagVisibility=global
  From3 : From  Commented=on  GotoTag=tr_fi  TagVisibility=global
  From30 : From  Commented=on  GotoTag=see_flag  TagVisibility=global
  From31 : From  Commented=on  GotoTag=tr_la  TagVisibility=global
  From32 : From  Commented=on  GotoTag=R1  TagVisibility=global
  From33 : From  Commented=on  GotoTag=pos_z_dgsk  TagVisibility=global
  From34 : From  Commented=on  GotoTag=pos_y_dgsk  TagVisibility=global
  From35 : From  Commented=on  GotoTag=pos_x_dgsk  TagVisibility=global
  From36 : From  Commented=on  GotoTag=tr_Z_dgsk  TagVisibility=global
  From37 : From  Commented=on  GotoTag=tr_Y_dgsk  TagVisibility=global
  From38 : From  Commented=on  GotoTag=tr_X_dgsk  TagVisibility=global
  From39 : From  Commented=on  GotoTag=D  TagVisibility=global
  From4 : From  Commented=on  GotoTag=tr_H  TagVisibility=global
  From40 : From  Commented=on  GotoTag=tr_fi  TagVisibility=global
  From41 : From  Commented=on  GotoTag=tr_H  TagVisibility=global
  From42 : From  Commented=on  GotoTag=del_D_p  TagVisibility=global
  From46 : From  Commented=on  GotoTag=Omega_id_geogr  TagVisibility=global
  From5 : From  Commented=on  GotoTag=tr_la  TagVisibility=global
  From61 : From  Commented=on  GotoTag=D1  TagVisibility=global
  From63 : From  Commented=on  GotoTag=Z_b_g  TagVisibility=global
  Goto : Goto  Commented=on  GotoTag=H_b_g
  MATLAB Function : MATLAB Function  Commented=on  TreatAsAtomicUnit=on
  MATLAB Function1 : MATLAB Function  Commented=on  TreatAsAtomicUnit=on
  MATLAB Function2 : MATLAB Function  TreatAsAtomicUnit=on
  MATLAB Function3 : MATLAB Function  TreatAsAtomicUnit=on
  MATLAB Function4 : MATLAB Function  TreatAsAtomicUnit=on
  MATLAB Function5 : MATLAB Function  TreatAsAtomicUnit=on
  MATLAB Function6 : MATLAB Function  TreatAsAtomicUnit=on
  MATLAB Function7 : MATLAB Function  Commented=on  TreatAsAtomicUnit=on
  Memory : Memory  InitialCondition=P0_b_g  LinearizeMemory=on
  Memory1 : Memory  InitialCondition=X0_b_g
  Scope{,3..7,9..17} (15 alike) : Scope
  Scope1 : Scope  Commented=on
  Scope2 : Scope  NumInputPorts=2
  Scope8 : Scope  NumInputPorts=2
  Sum : Sum  Commented=on  Inputs=|+-
  Sum1 : Sum  Inputs=|+-
  Sum2 : Sum  Commented=on  Inputs=|+-
  Sum3 : Sum  Inputs=|+-
  To Workspace1 : ToWorkspace  Commented=on  VariableName=G_b_g  SaveFormat=Structure  SampleTime=-1
      settings: Save2DSignal=2-D array (concatenate along first dimension)
  To Workspace2 : ToWorkspace  Commented=on  VariableName=F_b_g  SaveFormat=Structure  SampleTime=-1
      settings: Save2DSignal=2-D array (concatenate along first dimension)
  To Workspace3 : ToWorkspace  Commented=on  VariableName=Rv_b_g  SaveFormat=Structure  SampleTime=-1
      settings: Save2DSignal=2-D array (concatenate along first dimension)
  To Workspace4 : ToWorkspace  Commented=on  VariableName=H_b_g  SaveFormat=Structure  SampleTime=-1
      settings: Save2DSignal=2-D array (concatenate along first dimension)
  To Workspace5 : ToWorkspace  Commented=on  VariableName=Q_W  SaveFormat=Structure  SampleTime=-1
      settings: Save2DSignal=2-D array (concatenate along first dimension)
  tag scope: PP_TCS_UKF=global, X_TCS_UKF=global, X_feedback_TCS_UKF=global
  wires:
  From46/1 -> MATLAB Function/17(Omega_id_geogr)
  Constant8/1 -> MATLAB Function/9(R_e2)
  From34/1 -> MATLAB Function/12(pos_y_dgks)
  MATLAB Function/1(H_b_g) -> To Workspace4/1, Goto/1
  From24/1 -> MATLAB Function/7(ro2)
  From38/1 -> MATLAB Function/14(b_X_dgsk)
  From25/1 -> MATLAB Function/6(ro1)
  From37/1 -> MATLAB Function/15(b_Y_dgsk)
  From35/1 -> MATLAB Function/11(pos_x_dgks)
  From33/1 -> MATLAB Function/13(pos_z_dgks)
  From2/1 -> MATLAB Function/10(b_D_p)
  From36/1 -> MATLAB Function/16(b_Z_dgsk)
  From32/1 -> MATLAB Function/5(R1)
  Constant7/1 -> MATLAB Function/8(R_a)
  [F_b] -> MATLAB Function3/1(F_b)
  [G_b] -> MATLAB Function3/2(G_b)
  Constant2/1 -> MATLAB Function4/8(dt)
  Constant9/1 -> MATLAB Function5/1(sigma_error_D_p)
  Constant10/1 -> MATLAB Function5/2(sigma_error_D_p1)
  [sigma_DUS] -> MATLAB Function5/3(sigma_error_DUS)
  [sigma_acs] -> MATLAB Function5/4(sigma_error_acs)
  Constant3/1 -> MATLAB Function5/9(T), MATLAB Function5/8(dt)
  MATLAB Function3/1(F_b_g) -> [F_b_g], To Workspace2/1
  MATLAB Function4/1(P) -> Memory/1
  MATLAB Function3/2(G_b_g) -> To Workspace1/1, [G_b_g]
  MATLAB Function5/1(Rv_b_g) -> [Rv_b_g], To Workspace3/1
  MATLAB Function5/2(Q_W) -> To Workspace5/1, [Q_W]
  Memory1/1 -> MATLAB Function4/2("x ")
  Memory/1 -> MATLAB Function4/1("P ")
  Constant4/1 -> MATLAB Function5/5(SKO_gnss0)
  Constant5/1 -> MATLAB Function5/6(sigma_error_DUS0)
  Constant6/1 -> MATLAB Function5/7(sigma_error_acs0)
  From27/1 -> MATLAB Function/18(see_flag)
  Constant/1 -> MATLAB Function/19(al_gp_max)
  [see_flag] -> MATLAB Function5/10(see_flag)
  [X_b] -> Sum1/1, MATLAB Function6/1(X_b), MATLAB Function2/2(X_b)
  From3/1 -> MATLAB Function/2(tr_fi)
  From4/1 -> MATLAB Function/3(tr_H)
  From28/1 -> MATLAB Function/4(tr_V_H)
  From5/1 -> MATLAB Function/1(tr_la)
  MATLAB Function2/1(X_feedback) -> [X_feedback_TCS_UKF]
  MATLAB Function6/1(rate_X_feedback) -> Memory1/1
  [Q_W] -> MATLAB Function4/7(Q_km1)
  [Rv_b_g] -> MATLAB Function4/6(R_k)
  [G_b_g] -> MATLAB Function4/5(G)
  [F_b_g] -> MATLAB Function4/4(F)
  [Z_b_g] -> MATLAB Function4/3(z_k)
  MATLAB Function4/3(x_21) -> Sum1/2
  MATLAB Function4/2(x) -> Demux1/1, MATLAB Function6/2(rate_X)
  Sum1/1 -> Demux/1, [X_TCS_UKF], MATLAB Function2/1(X_diff)
  MATLAB Function4/5(x12) -> Scope3/1
  Constant12/1 -> MATLAB Function7/13(al_gp_max)
  From31/1 -> MATLAB Function7/7(tr_la)
  From13/1 -> MATLAB Function7/3(pos_y_dgsk)
  Constant11/1 -> MATLAB Function7/11(R_a)
  From40/1 -> MATLAB Function7/6(tr_fi)
  Constant13/1 -> MATLAB Function7/12(R_e2)
  From29/1 -> MATLAB Function7/2(pos_x_dgsk)
  From26/1 -> MATLAB Function7/14(D_p)
  From30/1 -> MATLAB Function7/5(see_flag)
  From11/1 -> MATLAB Function7/4(pos_z_dgsk)
  From14/1 -> MATLAB Function7/9(ro1)
  From41/1 -> MATLAB Function7/8(tr_H)
  From19/1 -> MATLAB Function7/10(ro2)
  From10/1 -> MATLAB Function7/1(rate_X)
  From42/1 -> MATLAB Function7/15(del_D_p)
  [pos_x_dgsk] -> MATLAB Function4/9(pos_x_dgsk)
  [pos_y_dgsk] -> MATLAB Function4/10(pos_y_dgsk)
  [pos_z_dgsk] -> MATLAB Function4/11(pos_z_dgsk)
  [see_flag] -> MATLAB Function4/15(see_flag)
  [tr_fi] -> MATLAB Function4/16(tr_fi)
  [tr_la] -> MATLAB Function4/17(tr_la)
  [tr_H] -> MATLAB Function4/18(tr_H)
  [ro1] -> MATLAB Function4/22(ro1)
  [ro2] -> MATLAB Function4/23(ro2)
  Constant14/1 -> MATLAB Function4/24(R_a)
  Constant16/1 -> MATLAB Function4/25(R_e2)
  Constant15/1 -> MATLAB Function4/26(al_gp_max)
  [D] -> MATLAB Function4/27(D_p)
  [vel_x_dgsk] -> MATLAB Function4/12(vel_x_dgsk)
  [vel_y_dgsk] -> MATLAB Function4/13(vel_y_dgsk)
  [vel_z_dgsk] -> MATLAB Function4/14(vel_z_dgsk)
  Constant17/1 -> MATLAB Function5/11(al_gp_max)
  [tr_V_H] -> MATLAB Function4/21(tr_V_H)
  [tr_V_N] -> MATLAB Function4/20(tr_V_N)
  [tr_V_E] -> MATLAB Function4/19(tr_V_E)
  [Omega_id_geogr] -> MATLAB Function4/28(Omega_id_geogr)
  [D1] -> MATLAB Function4/29(D1_p)
  Sum/1 -> Scope9/1
  From21/1 -> Sum/2
  MATLAB Function1/1(Z_b_g_) -> Sum/1
  From22/1 -> MATLAB Function1/1(rate_X)
  From23/1 -> MATLAB Function1/2(del_D_p)
  From39/1 -> MATLAB Function1/3(D_p)
  From61/1 -> MATLAB Function1/4(D1_p)
  Constant1/1 -> MATLAB Function1/5(al_gp_max)
  From63/1 -> Sum2/2
  Sum2/1 -> Scope1/1
  Demux2/17 -> Sum2/1
  MATLAB Function4/7(l) -> Sum3/1
  MATLAB Function4/6(e) -> Sum3/2, Scope2/1
  Sum3/1 -> Scope4/1
  Demux1/22 -> Scope8/1
  Demux1/23 -> Scope8/2
  Demux/1 -> Scope/1
  Demux/2 -> Scope11/1
  Demux/4 -> Scope10/1
  Demux/5 -> Scope12/1
  Demux1/2 -> Scope15/1
  Demux1/5 -> Scope5/1
  Demux1/4 -> Scope7/1
  Demux1/1 -> Scope6/1
  Demux2/1 -> Scope13/1
  Demux2/5 -> Scope17/1
  Demux2/2 -> Scope16/1
  Demux2/4 -> Scope14/1
  MATLAB Function4/4(PP) -> [PP_TCS_UKF], Demux2/1

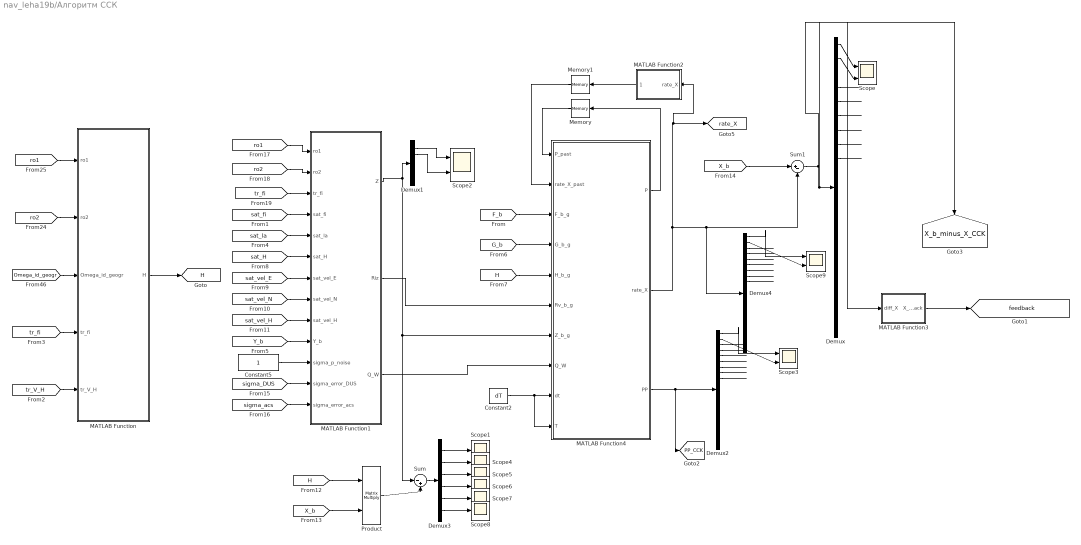
== system nav_leha19b/Алгоритм ССК ==
  Constant2 : Constant  Value=dT
  Constant5 : Constant
  Demux : Demux  Outputs=21
  Demux1 : Demux  Outputs=6
  Demux2 : Demux  Outputs=21
  Demux3 : Demux  Outputs=6
  Demux4 : Demux  Outputs=21
  MATLAB Function : MATLAB Function  TreatAsAtomicUnit=on
  MATLAB Function1 : MATLAB Function  TreatAsAtomicUnit=on
  MATLAB Function2 : MATLAB Function  TreatAsAtomicUnit=on
  MATLAB Function3 : MATLAB Function  TreatAsAtomicUnit=on
  MATLAB Function4 : MATLAB Function  TreatAsAtomicUnit=on
  Memory : Memory  InitialCondition=P_b
  Memory1 : Memory  InitialCondition=X0
  Product : Product  Multiplication=Matrix(*)
  Scope{,2..3,9} (4 alike) : Scope  NumInputPorts=2
  Scope{1,4..8} (6 alike) : Scope
  Sum : Sum  Inputs=|-+
  Sum1 : Sum  Inputs=|+-
  tag scope: H=global, PP_CCK=global, X_b_minus_X_CCK=global, feedback=global, rate_X=global
  wires:
  Constant2/1 -> MATLAB Function4/10(T), MATLAB Function4/9(dt)
  MATLAB Function4/1(P) -> Memory/1
  [F_b] -> MATLAB Function4/3(F_b_g)
  [G_b] -> MATLAB Function4/4(G_b_g)
  [H] -> MATLAB Function4/5(H_b_g)
  MATLAB Function4/2(rate_X) -> Demux4/1, Sum1/2, MATLAB Function2/1(rate_X), [rate_X]
  Memory1/1 -> MATLAB Function4/2(rate_X_past)
  Memory/1 -> MATLAB Function4/1(P_past)
  MATLAB Function4/3(PP) -> [PP_CCK], Demux2/1
  MATLAB Function/1(H) -> [H]
  [ro2] -> MATLAB Function/2(ro2)
  [ro1] -> MATLAB Function/1(ro1)
  [Omega_id_geogr] -> MATLAB Function/3(Omega_id_geogr)
  [tr_fi] -> MATLAB Function/4(tr_fi)
  [tr_V_H] -> MATLAB Function/5(tr_V_H)
  [Y_b] -> MATLAB Function1/10(Y_b)
  [sigma_DUS] -> MATLAB Function1/12(sigma_error_DUS)
  [sigma_acs] -> MATLAB Function1/13(sigma_error_acs)
  MATLAB Function1/1(Z) -> Demux1/1, Sum/1, MATLAB Function4/7(Z_b_g)
  MATLAB Function1/2(Riz) -> MATLAB Function4/6(Rv_b_g)
  MATLAB Function1/3(Q_W) -> MATLAB Function4/8(Q_W)
  [X_b] -> Sum1/1
  Sum1/1 -> MATLAB Function3/1(diff_X), Demux/1, [X_b_minus_X_CCK]
  [sat_fi] -> MATLAB Function1/4(sat_fi)
  [sat_la] -> MATLAB Function1/5(sat_la)
  [sat_H] -> MATLAB Function1/6(sat_H)
  [sat_vel_N] -> MATLAB Function1/8(sat_vel_N)
  [sat_vel_H] -> MATLAB Function1/9(sat_vel_H)
  [sat_vel_E] -> MATLAB Function1/7(sat_vel_E)
  Constant5/1 -> MATLAB Function1/11(sigma_p_noise)
  Demux1/1 -> Scope2/1
  Demux1/2 -> Scope2/2
  Demux/4 -> ?
  Demux/5 -> ?
  Demux/6 -> ?
  Demux/7 -> ?
  Demux/8 -> ?
  Demux/9 -> ?
  Demux2/1 -> Scope3/1
  Demux2/2 -> Scope3/2
  Demux2/3 -> ?
  Demux2/4 -> ?
  Demux2/5 -> ?
  Demux2/6 -> ?
  Demux2/7 -> ?
  Demux2/8 -> ?
  Demux2/9 -> ?
  Demux/1 -> Scope/1
  Demux/2 -> Scope/2
  Product/1 -> Sum/2
  [H] -> Product/1
  [X_b] -> Product/2
  Sum/1 -> Demux3/1
  Demux3/1 -> Scope1/1
  Demux3/2 -> Scope4/1
  Demux3/3 -> Scope5/1
  Demux3/4 -> Scope6/1
  Demux3/5 -> Scope7/1
  Demux3/6 -> Scope8/1
  [ro1] -> MATLAB Function1/1(ro1)
  [ro2] -> MATLAB Function1/2(ro2)
  Demux4/2 -> Scope9/2
  Demux4/6 -> ?
  Demux4/3 -> ?
  Demux4/5 -> ?
  Demux4/7 -> ?
  Demux4/1 -> Scope9/1
  Demux4/8 -> ?
  Demux4/4 -> ?
  Demux4/9 -> ?
  [tr_fi] -> MATLAB Function1/3(tr_fi)
  MATLAB Function3/1(X_CCK_feedback) -> [feedback]
  MATLAB Function2/1(rate_X_) -> Memory1/1
